simulink model "singlcontact_control_smc_lqr_mydimes_reaction"  (R2024a)
settings: Solver=VariableStepAuto  StartTime=0.0  StopTime=10  FixedStep=0.001  RelTol=1e-3
values from neighbouring files (symbols this model uses):
  ankle_servo_kd = 8    [robotParametersCtrl_mydiem_block_zmp.m]    (also in robotParametersCtrl_quad_modify_mydiem.m; robotParametersCtrl_quad_modify_mydiem_reaction.m)
  ankle_servo_ki = 4    [robotParametersCtrl_mydiem_block_zmp.m]    (also in robotParametersCtrl_quad_modify_mydiem.m; robotParametersCtrl_quad_modify_mydiem_reaction.m)
  ankle_servo_kp = 20    [robotParametersCtrl_mydiem_block_zmp.m]    (also in robotParametersCtrl_quad_modify_mydiem.m; robotParametersCtrl_quad_modify_mydiem_reaction.m)
  deriv_filter_coeff = 100    [robotParametersCtrl_mydiem_block_zmp.m]    (also in robotParametersCtrl_quad_modify_mydiem.m; robotParametersCtrl_quad_modify_mydiem_reaction.m)
  filter_coefficent_pid = 100    [robotParametersCtrl_mydiem_block_zmp.m]    (also in robotParametersCtrl_quad_modify_mydiem.m; robotParametersCtrl_quad_modify_mydiem_reaction.m)
  filter_coefficent_pids = 100    [robotParametersCtrl_quad_modify_mydiem_reaction.m]
  foot_z = 1.5    [robotParametersCtrl_mydiem_block_zmp.m]    (also in robotParametersCtrl_quad_modify_mydiem.m; robotParametersCtrl_quad_modify_mydiem_reaction.m)
  g = 9.81    [ABCDvalues_lqr_quad_mydime_reaction.m]    (also in robotParametersCtrl_mydiem_block_zmp.m = 9.80665; robotParametersCtrl_quad_modify_mydiem.m = 9.80665; robotParametersCtrl_quad_modify_mydiem_reaction.m = 9.80665)
  h = 32    [robotParametersCtrl_mydiem_block_zmp.m]    (also in robotParametersCtrl_quad_modify_mydiem.m; robotParametersCtrl_quad_modify_mydiem_reaction.m)
  height_plane = 0.025    [robotParametersCtrl_mydiem_block_zmp.m]    (also in robotParametersCtrl_quad_modify_mydiem.m; robotParametersCtrl_quad_modify_mydiem_reaction.m)
  hip_pitch_deriv = 20    [robotParametersCtrl_mydiem_block_zmp.m]    (also in robotParametersCtrl_quad_modify_mydiem.m = 200; robotParametersCtrl_quad_modify_mydiem_reaction.m = 200)
  hip_pitch_derivs = 200    [robotParametersCtrl_quad_modify_mydiem_reaction.m]
  hip_pitch_int = 0    [robotParametersCtrl_mydiem_block_zmp.m]    (also in robotParametersCtrl_quad_modify_mydiem.m = 150; robotParametersCtrl_quad_modify_mydiem_reaction.m = 150)
  hip_pitch_ints = 1500    [robotParametersCtrl_quad_modify_mydiem_reaction.m]
  hip_pitch_prop = 10    [robotParametersCtrl_mydiem_block_zmp.m]    (also in robotParametersCtrl_quad_modify_mydiem.m = 500; robotParametersCtrl_quad_modify_mydiem_reaction.m = 500)
  hip_pitch_props = 500    [robotParametersCtrl_quad_modify_mydiem_reaction.m]
  hip_roll_deriv = 28    [robotParametersCtrl_mydiem_block_zmp.m]    (also in robotParametersCtrl_quad_modify_mydiem.m = 280; robotParametersCtrl_quad_modify_mydiem_reaction.m = 280)
  hip_roll_derivs = 280    [robotParametersCtrl_quad_modify_mydiem_reaction.m]
  hip_roll_int = 0    [robotParametersCtrl_mydiem_block_zmp.m]    (also in robotParametersCtrl_quad_modify_mydiem.m = 180; robotParametersCtrl_quad_modify_mydiem_reaction.m = 180)
  hip_roll_ints = 180    [robotParametersCtrl_quad_modify_mydiem_reaction.m]
  hip_roll_prop = 10    [robotParametersCtrl_mydiem_block_zmp.m]    (also in robotParametersCtrl_quad_modify_mydiem.m = 300; robotParametersCtrl_quad_modify_mydiem_reaction.m = 300)
  hip_roll_props = 300    [robotParametersCtrl_quad_modify_mydiem_reaction.m]
  hip_servo_kd = 20    [robotParametersCtrl_mydiem_block_zmp.m]    (also in robotParametersCtrl_quad_modify_mydiem.m; robotParametersCtrl_quad_modify_mydiem_reaction.m)
  hip_servo_ki = 10    [robotParametersCtrl_mydiem_block_zmp.m]    (also in robotParametersCtrl_quad_modify_mydiem.m; robotParametersCtrl_quad_modify_mydiem_reaction.m)
  hip_servo_kp = 60    [robotParametersCtrl_mydiem_block_zmp.m]    (also in robotParametersCtrl_quad_modify_mydiem.m; robotParametersCtrl_quad_modify_mydiem_reaction.m)
  hip_smc_lamda = 85    [robotParametersCtrl_mydiem_block_zmp.m]    (also in robotParametersCtrl_quad_modify_mydiem.m; robotParametersCtrl_quad_modify_mydiem_reaction.m = 95)
  hip_smc_lamdas = 85    [robotParametersCtrl_quad_modify_mydiem_reaction.m]
  hip_smc_new = 25    [robotParametersCtrl_mydiem_block_zmp.m]    (also in robotParametersCtrl_quad_modify_mydiem.m; robotParametersCtrl_quad_modify_mydiem_reaction.m = 45)
  hip_smc_news = 25    [robotParametersCtrl_quad_modify_mydiem_reaction.m]
  init_angs_L = init_angs_R    [robotParametersCtrl_mydiem_block_zmp.m]    (also in robotParametersCtrl_quad_modify_mydiem.m; robotParametersCtrl_quad_modify_mydiem_reaction.m)
  init_angs_R = [0 -sum(init_angs) init_angs(2) 0 init_angs(1)]    [robotParametersCtrl_mydiem_block_zmp.m]    (also in robotParametersCtrl_quad_modify_mydiem.m; robotParametersCtrl_quad_modify_mydiem_reaction.m)
  init_height = h +                torso_z/2 + torso_offset_z + height_plane/2    (= 39.5125)    [robotParametersCtrl_mydiem_block_zmp.m]    (also in robotParametersCtrl_quad_modify_mydiem.m; robotParametersCtrl_quad_modify_mydiem_reaction.m)
  K = lqr(A, B, Q, R)    [ABCDvalues_lqr_quad_mydime_reaction.m]
  knee_pitch_deriv = 10    [robotParametersCtrl_mydiem_block_zmp.m]    (also in robotParametersCtrl_quad_modify_mydiem.m = 100; robotParametersCtrl_quad_modify_mydiem_reaction.m = 100)
  knee_pitch_derivs = 180    [robotParametersCtrl_quad_modify_mydiem_reaction.m]
  knee_pitch_int = 0    [robotParametersCtrl_mydiem_block_zmp.m]    (also in robotParametersCtrl_quad_modify_mydiem.m = 300; robotParametersCtrl_quad_modify_mydiem_reaction.m = 300)
  knee_pitch_ints = 7500    [robotParametersCtrl_quad_modify_mydiem_reaction.m]
  knee_pitch_prop = 10    [robotParametersCtrl_mydiem_block_zmp.m]    (also in robotParametersCtrl_quad_modify_mydiem.m = 400; robotParametersCtrl_quad_modify_mydiem_reaction.m = 400)
  knee_pitch_props = 1200    [robotParametersCtrl_quad_modify_mydiem_reaction.m]
  knee_servo_kd = 10    [robotParametersCtrl_mydiem_block_zmp.m]    (also in robotParametersCtrl_quad_modify_mydiem.m; robotParametersCtrl_quad_modify_mydiem_reaction.m)
  knee_servo_ki = 5    [robotParametersCtrl_mydiem_block_zmp.m]    (also in robotParametersCtrl_quad_modify_mydiem.m; robotParametersCtrl_quad_modify_mydiem_reaction.m)
  knee_servo_kp = 60    [robotParametersCtrl_mydiem_block_zmp.m]    (also in robotParametersCtrl_quad_modify_mydiem.m; robotParametersCtrl_quad_modify_mydiem_reaction.m)
  knee_smc_lamda = 140    [robotParametersCtrl_mydiem_block_zmp.m]    (also in robotParametersCtrl_quad_modify_mydiem.m; robotParametersCtrl_quad_modify_mydiem_reaction.m = 150)
  knee_smc_lamdas = 100    [robotParametersCtrl_quad_modify_mydiem_reaction.m]
  knee_smc_new = 80    [robotParametersCtrl_mydiem_block_zmp.m]    (also in robotParametersCtrl_quad_modify_mydiem.m; robotParametersCtrl_quad_modify_mydiem_reaction.m)
  knee_smc_news = 60    [robotParametersCtrl_quad_modify_mydiem_reaction.m]
  Kwalk = 0.6    [robotParametersCtrl_mydiem_block_zmp.m]    (also in robotParametersCtrl_quad_modify_mydiem.m; robotParametersCtrl_quad_modify_mydiem_reaction.m)
  l1 = 0.20    (= 0.2)    [ABCDvalues_lqr_quad_mydime_reaction.m]
  l2 = 0.20    (= 0.2)    [ABCDvalues_lqr_quad_mydime_reaction.m]
  lower_leg_length = 20    [robotParametersCtrl_mydiem_block_zmp.m]    (also in robotParametersCtrl_quad_modify_mydiem.m; robotParametersCtrl_quad_modify_mydiem_reaction.m)
  m1 = 0.45    [ABCDvalues_lqr_quad_mydime_reaction.m]
  m2 = 0.065    [ABCDvalues_lqr_quad_mydime_reaction.m]
  max_torque = 20    [robotParametersCtrl_mydiem_block_zmp.m]    (also in robotParametersCtrl_quad_modify_mydiem.m; robotParametersCtrl_quad_modify_mydiem_reaction.m)
  motion_time_constant = 0.01    [robotParametersCtrl_mydiem_block_zmp.m]    (also in robotParametersCtrl_quad_modify_mydiem.m; robotParametersCtrl_quad_modify_mydiem_reaction.m)
  plane_x = 25    [robotParametersCtrl_mydiem_block_zmp.m]    (also in robotParametersCtrl_quad_modify_mydiem.m; robotParametersCtrl_quad_modify_mydiem_reaction.m)
  plane_y = 3    [robotParametersCtrl_mydiem_block_zmp.m]    (also in robotParametersCtrl_quad_modify_mydiem.m; robotParametersCtrl_quad_modify_mydiem_reaction.m)
  stepHeight = 0.4    [ABCDvalues_lqr_quad_mydime_reaction.m]
  torso_offset_x = 17    [robotParametersCtrl_mydiem_block_zmp.m]    (also in robotParametersCtrl_quad_modify_mydiem.m; robotParametersCtrl_quad_modify_mydiem_reaction.m)
  torso_offset_x1 = -17    [robotParametersCtrl_mydiem_block_zmp.m]    (also in robotParametersCtrl_quad_modify_mydiem.m; robotParametersCtrl_quad_modify_mydiem_reaction.m)
  torso_offset_z = 0    [robotParametersCtrl_mydiem_block_zmp.m]    (also in robotParametersCtrl_quad_modify_mydiem.m; robotParametersCtrl_quad_modify_mydiem_reaction.m)
  torso_x = 40    [robotParametersCtrl_mydiem_block_zmp.m]    (also in robotParametersCtrl_quad_modify_mydiem.m; robotParametersCtrl_quad_modify_mydiem_reaction.m)
  torso_y = 20    [robotParametersCtrl_mydiem_block_zmp.m]    (also in robotParametersCtrl_quad_modify_mydiem.m; robotParametersCtrl_quad_modify_mydiem_reaction.m)
  torso_z = 15    [robotParametersCtrl_mydiem_block_zmp.m]    (also in robotParametersCtrl_quad_modify_mydiem.m; robotParametersCtrl_quad_modify_mydiem_reaction.m)
  Ts = 0.05    [ABCDvalues_lqr_quad_mydime_reaction.m]
  TsCtrl = 0.05    [robotParametersCtrl_mydiem_block_zmp.m]    (also in robotParametersCtrl_quad_modify_mydiem.m; robotParametersCtrl_quad_modify_mydiem_reaction.m)
  tWalk = 0.3    [robotParametersCtrl_mydiem_block_zmp.m]    (also in robotParametersCtrl_quad_modify_mydiem.m; robotParametersCtrl_quad_modify_mydiem_reaction.m)
  upper_leg_length = 20    [robotParametersCtrl_mydiem_block_zmp.m]    (also in robotParametersCtrl_quad_modify_mydiem.m; robotParametersCtrl_quad_modify_mydiem_reaction.m)
undefined symbols (not defined in the file or in its folder): X, Y, Z
libraries: simulink_extras x256, slpidlib x128, sm_lib x71, simulink x43, nesl_utility x35, walkingRobotUtils x21, dspsrcs4 x18, dspobslib x8
(part 1 of 33)
settings Model: Creator=sunil kumar  LastModifiedBy=USER
settings OptimizationCC: BlockReduction=off  DefaultParameterBehavior=Inlined  BufferReuse=off
settings RTWCC: GPUComputeCapability=3.5

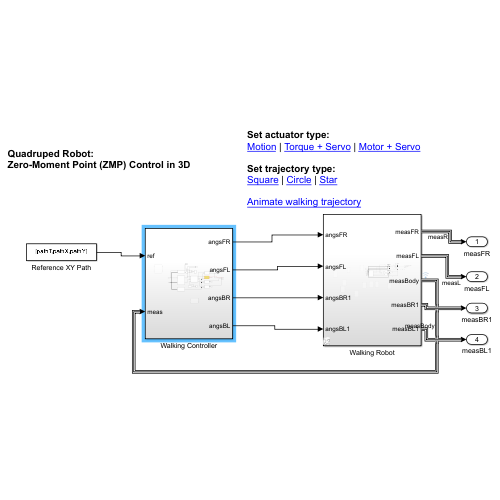
[thumbnail: Simulink's stored preview of the top-level diagram]
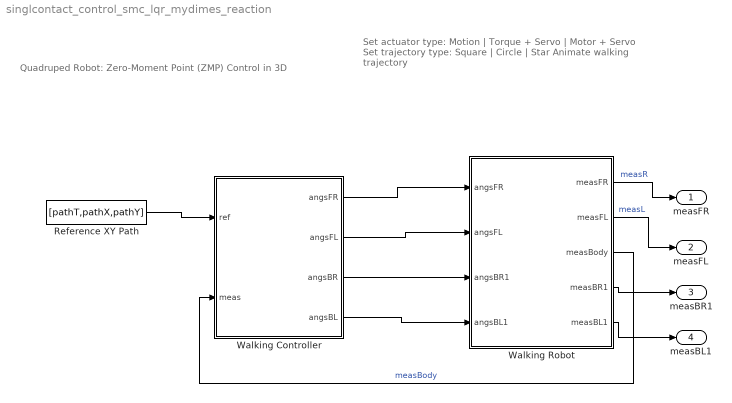
== system singlcontact_control_smc_lqr_mydimes_reaction ==
  note: Set actuator type:
      | Motion | Torque + Servo | Motor + Servo
      |
      | Set trajectory type:
      | Square | Circle | Star
      |
      | Animate walking trajectory
  note: Quadruped Robot:
      | Zero-Moment Point (ZMP) Control in 3D
  Reference XY Path : FromWorkspace  VariableName=[pathT,pathX,pathY]  SampleTime=TsCtrl  OutputAfterFinalValue=Holding final value
  Walking Controller : Subsystem
  Walking Robot : Subsystem  AncestorBlock=|
      | walkingRobotUtils/Walking Robot
      | (Control Design)
  measFR : Outport  VectorParamsAs1DForOutWhenUnconnected=off
  measFL : Outport  Port=2  VectorParamsAs1DForOutWhenUnconnected=off
  measBR1 : Outport  Port=3  VectorParamsAs1DForOutWhenUnconnected=off
  measBL1 : Outport  Port=4  VectorParamsAs1DForOutWhenUnconnected=off
  wires:
  Reference XY Path/1 -> Walking Controller/1(ref)
  Walking Robot/2(measFL) -> measFL/1  "measL"
  Walking Robot/1(measFR) -> measFR/1  "measR"
  Walking Controller/1(angsFR) -> Walking Robot/1(angsFR)
  Walking Controller/2(angsFL) -> Walking Robot/2(angsFL)
  Walking Robot/3(measBody) -> Walking Controller/2(meas)  "measBody"
  Walking Controller/3(angsBR) -> Walking Robot/3(angsBR1)
  Walking Controller/4(angsBL) -> Walking Robot/4(angsBL1)
  Walking Robot/4(measBR1) -> measBR1/1
  Walking Robot/5(measBL1) -> measBL1/1

== system singlcontact_control_smc_lqr_mydimes_reaction/Walking Controller ==
  ref : Inport
  meas : Inport  Port=2
  Calculate Attitude : Subsystem
  Digital Clock : DigitalClock  SampleTime=0.05
  Left Leg Inverse Kinematics : walkingRobotUtils/Inverse Kinematics (Control Design)  SystemSampleTime=-1  VariantActivationTime=update diagram  AllowFlexibleInterface=on  Latency=0  AutoFrameSizeCalculation=off
  Left Leg Inverse Kinematics1 : walkingRobotUtils/Inverse Kinematics (Control Design)  SystemSampleTime=-1  VariantActivationTime=update diagram  AllowFlexibleInterface=on  Latency=0  AutoFrameSizeCalculation=off
  Mux : Mux  Inputs=2
  Package Signals : Subsystem
  Position1 : Scope
  Right Leg Inverse Kinematics : walkingRobotUtils/Inverse Kinematics (Control Design)  SystemSampleTime=-1  VariantActivationTime=update diagram  AllowFlexibleInterface=on  Latency=0  AutoFrameSizeCalculation=off
  Right Leg Inverse Kinematics1 : walkingRobotUtils/Inverse Kinematics (Control Design)  SystemSampleTime=-1  VariantActivationTime=update diagram  AllowFlexibleInterface=on  Latency=0  AutoFrameSizeCalculation=off
  Scope : Scope  NumInputPorts=2
  Scope1 : Scope  NumInputPorts=4
  Scope2 : Scope
  Scope3 : Scope  NumInputPorts=2
  Step Planning Logic : Stateflow chart  Commented=on  TreatAsAtomicUnit=on
  ZMP Controller : Subsystem
  Zero-Order Hold : ZeroOrderHold  SampleTime=0.005
  final logic working quad_trot : MATLAB Function  TreatAsAtomicUnit=on
  final logic working quad_walk1 : MATLAB Function  Commented=on  TreatAsAtomicUnit=on
  angsFR : Outport  VectorParamsAs1DForOutWhenUnconnected=off
  angsFL : Outport  Port=2  VectorParamsAs1DForOutWhenUnconnected=off
  angsBR : Outport  Port=3  VectorParamsAs1DForOutWhenUnconnected=off
  angsBL : Outport  Port=4  VectorParamsAs1DForOutWhenUnconnected=off
  wires:
  ref/1 -> ZMP Controller/1(ref), Package Signals/1(ref)
  Right Leg Inverse Kinematics/1 -> Scope1/1, angsFR/1
  Left Leg Inverse Kinematics/1 -> Scope1/3, angsFL/1
  meas/1 -> Calculate Attitude/1(meas), Package Signals/2(meas), ZMP Controller/2("meas ")
  Package Signals/2(y) -> Zero-Order Hold/1  "Y"
  Package Signals/1(x) -> Scope3/1, Mux/1  "X"
  Calculate Attitude/1(att) -> Left Leg Inverse Kinematics/2, Right Leg Inverse Kinematics1/2, Right Leg Inverse Kinematics/2, Left Leg Inverse Kinematics1/2
  Digital Clock/1 -> final logic working quad_trot/3(timeElapsed), Scope2/1
  final logic working quad_trot/1(footFR) -> Right Leg Inverse Kinematics/1
  ZMP Controller/1(stepFwd) -> final logic working quad_trot/1(stepFwd), Scope/1
  ZMP Controller/2(stepLat) -> final logic working quad_trot/2(stepLat), Scope/2
  final logic working quad_trot/2(footFL) -> Left Leg Inverse Kinematics/1  "L"
  final logic working quad_trot/4(footBL) -> Left Leg Inverse Kinematics1/1
  final logic working quad_trot/3(footBR) -> Right Leg Inverse Kinematics1/1
  Right Leg Inverse Kinematics1/1 -> Scope1/2, angsBR/1
  Left Leg Inverse Kinematics1/1 -> Scope1/4, angsBL/1
  Zero-Order Hold/1 -> Scope3/2, Mux/2
  Mux/1 -> Position1/1

== system singlcontact_control_smc_lqr_mydimes_reaction/Walking Robot ==
  angsFR : Inport
  angsFL : Inport  Port=2
  angsBR1 : Inport  Port=3
  angsBL1 : Inport  Port=4
  6-DOF Joint : sm_lib/Joints/6-DOF Joint  JointMode=Normal  CompositeWrenchDir=FollowerOnBase  CompositeWrenchFrame=BaseFrame  SenseConstraintForce=off  SenseConstraintTorque=off  SenseTotalForce=off  SenseTotalTorque=off  PxPositionTargetSpecify=on  PxPositionTargetPriority=High  PxPositionTargetValue=0  PxPositionTargetValueUnits=m  PxVelocityTargetSpecify=off  PxVelocityTargetPriority=High  PxVelocityTargetValue=0  PxVelocityTargetValueUnits=m/s  PxEquilibriumPosition=0  PxEquilibriumPositionUnits=m  PxSpringStiffness=0  PxSpringStiffnessUnits=N/m  PxDampingCoefficient=world_damping  PxDampingCoefficientUnits=N/(m/s)  PxLowerLimitSpecify=off  PxLowerLimitBound=-1  PxLowerLimitBoundUnits=m  PxLowerLimitStiffness=1e6  PxLowerLimitStiffnessUnits=N/m  PxLowerLimitDamping=1e3  PxLowerLimitDampingUnits=N/(m/s)  PxLowerLimitTransitionRegionWidth=1e-4  PxLowerLimitTransitionRegionWidthUnits=m  PxUpperLimitSpecify=off  PxUpperLimitBound=1  PxUpperLimitBoundUnits=m  PxUpperLimitStiffness=1e6  PxUpperLimitStiffnessUnits=N/m  PxUpperLimitDamping=1e3  PxUpperLimitDampingUnits=N/(m/s)  PxUpperLimitTransitionRegionWidth=1e-4  PxUpperLimitTransitionRegionWidthUnits=m  PxTorqueActuationMode=NoTorque  PxMotionActuationMode=ComputedMotion  PxSensePosition=off  PxSenseVelocity=off  PxSenseAcceleration=off  PxSenseTorqueForce=off  PxSenseLowerLimitTorqueForce=off  PxSenseUpperLimitTorqueForce=off  PyPositionTargetSpecify=on  PyPositionTargetPriority=High  PyPositionTargetValue=0  PyPositionTargetValueUnits=m  PyVelocityTargetSpecify=off  PyVelocityTargetPriority=High  PyVelocityTargetValue=0  PyVelocityTargetValueUnits=m/s  PyEquilibriumPosition=0  PyEquilibriumPositionUnits=m  PySpringStiffness=0  PySpringStiffnessUnits=N/m  PyDampingCoefficient=world_damping  PyDampingCoefficientUnits=N/(m/s)  PyLowerLimitSpecify=off  PyLowerLimitBound=-1  PyLowerLimitBoundUnits=m  PyLowerLimitStiffness=1e6  PyLowerLimitStiffnessUnits=N/m  PyLowerLimitDamping=1e3  PyLowerLimitDampingUnits=N/(m/s)  PyLowerLimitTransitionRegionWidth=1e-4  PyLowerLimitTransitionRegionWidthUnits=m  PyUpperLimitSpecify=off  PyUpperLimitBound=1  PyUpperLimitBoundUnits=m  PyUpperLimitStiffness=1e6  PyUpperLimitStiffnessUnits=N/m  PyUpperLimitDamping=1e3  PyUpperLimitDampingUnits=N/(m/s)  PyUpperLimitTransitionRegionWidth=1e-4  PyUpperLimitTransitionRegionWidthUnits=m  PyTorqueActuationMode=NoTorque  PyMotionActuationMode=ComputedMotion  PySensePosition=off  PySenseVelocity=off  PySenseAcceleration=off  PySenseTorqueForce=off  PySenseLowerLimitTorqueForce=off  PySenseUpperLimitTorqueForce=off  PzPositionTargetSpecify=on  PzPositionTargetPriority=High  PzPositionTargetValue=init_height  PzPositionTargetValueUnits=cm  PzVelocityTargetSpecify=off  PzVelocityTargetPriority=High  PzVelocityTargetValue=0  PzVelocityTargetValueUnits=m/s  PzEquilibriumPosition=0  PzEquilibriumPositionUnits=m  PzSpringStiffness=0  PzSpringStiffnessUnits=N/m  PzDampingCoefficient=world_damping  PzDampingCoefficientUnits=N/(m/s)  PzLowerLimitSpecify=off  PzLowerLimitBound=-1  PzLowerLimitBoundUnits=m  PzLowerLimitStiffness=1e6  PzLowerLimitStiffnessUnits=N/m  PzLowerLimitDamping=1e3  PzLowerLimitDampingUnits=N/(m/s)  PzLowerLimitTransitionRegionWidth=1e-4  PzLowerLimitTransitionRegionWidthUnits=m  PzUpperLimitSpecify=off  PzUpperLimitBound=1  PzUpperLimitBoundUnits=m  PzUpperLimitStiffness=1e6  PzUpperLimitStiffnessUnits=N/m  PzUpperLimitDamping=1e3  PzUpperLimitDampingUnits=N/(m/s)  PzUpperLimitTransitionRegionWidth=1e-4  PzUpperLimitTransitionRegionWidthUnits=m  PzTorqueActuationMode=NoTorque  PzMotionActuationMode=ComputedMotion  PzSensePosition=off  PzSenseVelocity=off  PzSenseAcceleration=off  PzSenseTorqueForce=off  PzSenseLowerLimitTorqueForce=off  PzSenseUpperLimitTorqueForce=off  SphPositionTargetSpecify=off  SphPositionTargetPriority=High  SphPositionTargetRotationMethod=None  SphPositionTargetFollAlignAxisA=+X  SphPositionTargetBaseAlignAxisA=+Y  SphPositionTargetFollAlignAxisB=+Y  SphPositionTargetBaseAlignAxisB=+Z  SphPositionTargetRotationStandardAxis=+Z  SphPositionTargetRotationAngle=0.0  SphPositionTargetRotationAngleUnits=deg  SphPositionTargetRotationArbitraryAxis=[0 0 1]  SphPositionTargetRotationSequenceAxes=FollowerAxes  SphPositionTargetRotationSequence=XYX  SphPositionTargetRotationSequenceAngles=[0 0 0]  SphPositionTargetRotationSequenceAnglesUnits=deg  SphPositionTargetRotationMatrix=eye(3)  SphPositionTargetQuaternion=[1 0 0 0]  SphVelocityTargetSpecify=off  SphVelocityTargetPriority=High  SphVelocityTargetValue=[0 0 0]  SphVelocityTargetValueUnits=deg/s  SphVelocityTargetInFollowerFrame=on  SphEqPosRotationMethod=None  SphEqPosFollAlignAxisA=+X  SphEqPosBaseAlignAxisA=+Y  SphEqPosFollAlignAxisB=+Y  SphEqPosBaseAlignAxisB=+Z  SphEqPosRotationStandardAxis=+Z  SphEqPosRotationAngle=0.0  SphEqPosRotationAngleUnits=deg  SphEqPosRotationArbitraryAxis=[0 0 1]  SphEqPosRotationSequenceAxes=FollowerAxes  SphEqPosRotationSequence=XYX  SphEqPosRotationSequenceAngles=[0 0 0]  SphEqPosRotationSequenceAnglesUnits=deg  SphEqPosRotationMatrix=[1 0 0; 0 1 0; 0 0 1]  SphEqPosQuaternion=[1 0 0 0]  SphSpringStiffness=0  SphSpringStiffnessUnits=N*m/deg  SphDampingCoefficient=world_rot_damping  SphDampingCoefficientUnits=N*m/(rad/s)  SphLowerLimitSpecify=off  SphLowerLimitBound=15  SphLowerLimitBoundUnits=deg  SphLowerLimitStiffness=1e4  SphLowerLimitStiffnessUnits=N*m/deg  SphLowerLimitDamping=10  SphLowerLimitDampingUnits=N*m/(deg/s)  SphLowerLimitTransitionRegionWidth=0.1  SphLowerLimitTransitionRegionWidthUnits=deg  SphUpperLimitSpecify=off  SphUpperLimitBound=45  SphUpperLimitBoundUnits=deg  SphUpperLimitStiffness=1e4  SphUpperLimitStiffnessUnits=N*m/deg  SphUpperLimitDamping=10  SphUpperLimitDampingUnits=N*m/(deg/s)  SphUpperLimitTransitionRegionWidth=0.1  SphUpperLimitTransitionRegionWidthUnits=deg  SphTorqueActuationMode=NoTorque  SphActuateTorqueX=off  SphActuateTorqueY=off  SphActuateTorqueZ=off  SphActuateTorque=off  SphActuationFrame=BaseFrame  SphSensePosition=off  SphSenseVelocityX=off  SphSenseVelocityY=off  SphSenseVelocityZ=off  SphSenseVelocity=off  SphSenseAccelerationX=off  SphSenseAccelerationY=off  SphSenseAccelerationZ=off  SphSenseAcceleration=off  SphSenseLowerLimitTorqueMag=off  SphSenseUpperLimitTorqueMag=off  SphSensingFrame=BaseFrame
  Left Hip to Torso : sm_lib/Frames and Transforms/Rigid Transform  RotationMethod=None  FollAlignAxisA=+X  BaseAlignAxisA=+Y  FollAlignAxisB=+Y  BaseAlignAxisB=+Z  RotationStandardAxis=+Z  RotationAngle=0.0  RotationAngleUnits=deg  RotationArbitraryAxis=[0 0 1]  RotationSequenceAxes=FollowerAxes  RotationSequence=XYX  RotationSequenceAngles=[0 0 0]  RotationSequenceAnglesUnits=deg  RotationMatrix=[1 0 0; 0 1 0; 0 0 1]  Quaternion=[1 0 0 0]  TranslationMethod=Cartesian  TranslationCartesianOffset=[torso_offset_x torso_y/2 torso_offset_z]  TranslationCartesianOffsetUnits=cm  TranslationStandardAxis=+Z  TranslationStandardOffset=0  TranslationStandardOffsetUnits=cm  TranslationROffset=0  TranslationROffsetUnits=m  TranslationThetaOffset=0  TranslationThetaOffsetUnits=deg  TranslationZOffset=0  TranslationZOffsetUnits=m
  Left Hip to Torso1 : sm_lib/Frames and Transforms/Rigid Transform  RotationMethod=None  FollAlignAxisA=+X  BaseAlignAxisA=+Y  FollAlignAxisB=+Y  BaseAlignAxisB=+Z  RotationStandardAxis=+Z  RotationAngle=0.0  RotationAngleUnits=deg  RotationArbitraryAxis=[0 0 1]  RotationSequenceAxes=FollowerAxes  RotationSequence=XYX  RotationSequenceAngles=[0 0 0]  RotationSequenceAnglesUnits=deg  RotationMatrix=[1 0 0; 0 1 0; 0 0 1]  Quaternion=[1 0 0 0]  TranslationMethod=Cartesian  TranslationCartesianOffset=[torso_offset_x1 torso_y/2 torso_offset_z]  TranslationCartesianOffsetUnits=cm  TranslationStandardAxis=+Z  TranslationStandardOffset=0  TranslationStandardOffsetUnits=cm  TranslationROffset=0  TranslationROffsetUnits=m  TranslationThetaOffset=0  TranslationThetaOffsetUnits=deg  TranslationZOffset=0  TranslationZOffsetUnits=m
  Lqr+Lqr+reaction : Subsystem  Commented=on  VariantControl=actuatorType == 1
  NO CONTROLLER : Subsystem  Commented=on  VariantControl=actuatorType == 1
  PS-Simulink Converter : nesl_utility/PS-Simulink Converter  PhysicalDomain=network_engine_domain  SubClassName=ps_output  LeftPortType=input  RightPortType=output  PseudoPeriodic=off  Frequencies=[]  VectorFormat=inherit  Unit=inherit  AffineConversion=off
  PS-Simulink Converter1 : nesl_utility/PS-Simulink Converter  PhysicalDomain=network_engine_domain  SubClassName=ps_output  LeftPortType=input  RightPortType=output  PseudoPeriodic=off  Frequencies=[]  VectorFormat=inherit  Unit=inherit  AffineConversion=off
  PS-Simulink Converter2 : nesl_utility/PS-Simulink Converter  PhysicalDomain=network_engine_domain  SubClassName=ps_output  LeftPortType=input  RightPortType=output  PseudoPeriodic=off  Frequencies=[]  VectorFormat=inherit  Unit=inherit  AffineConversion=off
  Pid+Pid+reaction1 : Subsystem  Commented=on  VariantControl=actuatorType == 1
  Right Hip to Torso : sm_lib/Frames and Transforms/Rigid Transform  RotationMethod=None  FollAlignAxisA=+X  BaseAlignAxisA=+Y  FollAlignAxisB=+Y  BaseAlignAxisB=+Z  RotationStandardAxis=+Z  RotationAngle=0.0  RotationAngleUnits=deg  RotationArbitraryAxis=[0 0 1]  RotationSequenceAxes=FollowerAxes  RotationSequence=XYX  RotationSequenceAngles=[0 0 0]  RotationSequenceAnglesUnits=deg  RotationMatrix=[1 0 0; 0 1 0; 0 0 1]  Quaternion=[1 0 0 0]  TranslationMethod=Cartesian  TranslationCartesianOffset=[torso_offset_x -torso_y/2 torso_offset_z]  TranslationCartesianOffsetUnits=cm  TranslationStandardAxis=+Z  TranslationStandardOffset=0  TranslationStandardOffsetUnits=cm  TranslationROffset=0  TranslationROffsetUnits=m  TranslationThetaOffset=0  TranslationThetaOffsetUnits=deg  TranslationZOffset=0  TranslationZOffsetUnits=m
  Right Hip to Torso1 : sm_lib/Frames and Transforms/Rigid Transform  RotationMethod=None  FollAlignAxisA=+X  BaseAlignAxisA=+Y  FollAlignAxisB=+Y  BaseAlignAxisB=+Z  RotationStandardAxis=+Z  RotationAngle=0.0  RotationAngleUnits=deg  RotationArbitraryAxis=[0 0 1]  RotationSequenceAxes=FollowerAxes  RotationSequence=XYX  RotationSequenceAngles=[0 0 0]  RotationSequenceAnglesUnits=deg  RotationMatrix=[1 0 0; 0 1 0; 0 0 1]  Quaternion=[1 0 0 0]  TranslationMethod=Cartesian  TranslationCartesianOffset=[torso_offset_x1 -torso_y/2 torso_offset_z]  TranslationCartesianOffsetUnits=cm  TranslationStandardAxis=+Z  TranslationStandardOffset=0  TranslationStandardOffsetUnits=cm  TranslationROffset=0  TranslationROffsetUnits=m  TranslationThetaOffset=0  TranslationThetaOffsetUnits=deg  TranslationZOffset=0  TranslationZOffsetUnits=m
  Robot Joint Controller : Subsystem  Commented=on  Variant=on
  Robot Leg BL3 : Subsystem
  Robot Leg BR2 : Subsystem
  Robot Leg FL1 : Subsystem
  Robot Leg FR : Subsystem
  Scope : Scope  NumInputPorts=2
  Sensors : Subsystem
  Torso : sm_lib/Body Elements/Brick Solid  BrickDimensions=[torso_x torso_y torso_z]  BrickDimensionsUnits=cm  ExportEntireGeometry=off  InertiaType=PointMass  BasedOnType=Mass  Density=density  DensityUnits=kg/m^3  Mass=6  MassUnits=kg  CenterOfMass=[0 0 0]  CenterOfMassUnits=m  MomentsOfInertia=[1 1 1]  MomentsOfInertiaUnits=kg*m^2  ProductsOfInertia=[1 1 1]  ProductsOfInertiaUnits=kg*m^2  GraphicType=FromGeometry  MarkerShape=Sphere  MarkerSize=10  GraphicVisPropType=SimpleVisualProperties  GraphicDiffuseColor=[0.5 0.1 0.5]  GraphicOpacity=1.0  GraphicSpecularColor=[0.5 0.5 0.5 1.0]  GraphicAmbientColor=[0.15 0.15 0.15 1.0]  GraphicEmissiveColor=[0.0 0.0 0.0 1.0]  GraphicShininess=75  DoExposeReferenceFrame=on  SerializedFrames=<Frames><Frame><Id>Frame1</Id><Value><Name>F1</Name><Origin><Source>CenterOfMassFrame</Source><FeatureName></FeatureName></Origin><PrimaryAxis><DefinedDirection>+Z</DefinedDirection><Source>ReferenceFrame</Source><SourceDirection>+Z</SourceDirection><FeatureName></FeatureName></PrimaryAxis><SecondaryAxis><DefinedDirection>+Y</DefinedDirection><Source>ReferenceFrame</Source><SourceDirection>+X</SourceDirection><FeatureName></FeatureName></SecondaryAxis></Value></Frame></Frames>
  Torso2torso : sm_lib/Frames and Transforms/Rigid Transform  Commented=on  RotationMethod=None  FollAlignAxisA=+X  BaseAlignAxisA=+Y  FollAlignAxisB=+Y  BaseAlignAxisB=+Z  RotationStandardAxis=+Z  RotationAngle=0.0  RotationAngleUnits=deg  RotationArbitraryAxis=[0 0 1]  RotationSequenceAxes=FollowerAxes  RotationSequence=XYX  RotationSequenceAngles=[0 0 0]  RotationSequenceAnglesUnits=deg  RotationMatrix=[1 0 0; 0 1 0; 0 0 1]  Quaternion=[1 0 0 0]  TranslationMethod=Cartesian  TranslationCartesianOffset=[0 0 -7.5]  TranslationCartesianOffsetUnits=cm  TranslationStandardAxis=+Z  TranslationStandardOffset=0  TranslationStandardOffsetUnits=cm  TranslationROffset=0  TranslationROffsetUnits=m  TranslationThetaOffset=0  TranslationThetaOffsetUnits=deg  TranslationZOffset=0  TranslationZOffsetUnits=m
  Trajectory Display : sm_lib/Curves and Surfaces/Spline  DataPoints=interPts  DataPointsUnits=m  EndConditionType=Natural  GraphicType=FromGeometry  MarkerShape=Sphere  MarkerSize=10  GraphicVisPropType=SimpleVisualProperties  GraphicDiffuseColor=[0 0 0]  GraphicOpacity=1.0  GraphicSpecularColor=[0.5 0.5 0.5 1.0]  GraphicAmbientColor=[0.15 0.15 0.15 1.0]  GraphicEmissiveColor=[0.0 0.0 0.0 1.0]  GraphicShininess=75
  Transform Sensor : sm_lib/Frames and Transforms/Transform Sensor  MeasurementFrame=Base  RotationSequence=XYZ  SenseAngle=off  SenseAxis=off  SenseQ=off  SenseR=off  SenseRotationSequence=off  SenseOmegaX=off  SenseOmegaY=off  SenseOmegaZ=off  SenseOmega=off  SenseQDot=off  SenseRDot=off  SenseRotationSequenceDot=off  SenseAlphaX=off  SenseAlphaY=off  SenseAlphaZ=off  SenseAlpha=off  SenseQDDot=off  SenseRDDot=off  SenseX=on  SenseY=on  SenseZ=on  SenseXYZ=off  SenseRad=off  SenseAzim=off  SenseDist=off  SenseInc=off  SenseXDot=on  SenseYDot=off  SenseZDot=off  SenseXYZDot=off  SenseRadDot=off  SenseAzimDot=off  SenseDistDot=off  SenseIncDot=off  SenseXDDot=off  SenseYDDot=off  SenseZDDot=off  SenseXYZDDot=off  SenseRadDDot=off  SenseAzimDDot=off  SenseDistDDot=off  SenseIncDDot=off
  World and Ground : Subsystem
  XY Graph : Record  FileSettingsInternal="{\"entries\":[{\"content\":{\"excelSettings\":{\"content\":{},\"type\":\"Streamout.ExcelSettings\"}},\"type\":\"Streamout.FileSettingStorage\",\"uuid\":\"\"}],\"packageUris\":[\"http:\\/\\/schema.mathworks.com\\/mf0\\/streamout_blocks\\/R2020a\"],\"version\":\"1.0\"}"  Layout=[1 1]  SignalsInternal="{\"entries\":[{\"content\":{\"signals\":[{\"content\":{\"blockPath\":[],\"dimensions\":[1],\"domain\":\"\",\"lineColor\":\"#139fff\",\"lineWidth\":2,\"port\":1,\"sid\":[\"\"],\"signalID\":1,\"signalName\":\"PS-Simulink\\nConverter\"},\"type\":\"RecordBlkView.Signal\",\"uuid\":\"\"},{\"content\":{\"blockPath\":[],\"dimensions\":[1],\"domain\":\"\",\"lineColor\":\"#ff6929\",\"lineWidth\":2,\"port\":2,\"sid\":[\"\"],\"signalID\":2,\"signalName\":\"PS-Simulink\\nConverter1\"},\"type\":\"RecordBlkView.Signal\",\"uuid\":\"\"}]},\"type\":\"RecordBlkView.InputSignals\",\"uuid\":\"\"}],\"packageUris\":[\"http:\\/\\/schema.mathworks.com\\/mf0\\/streamout_blocks\\/R2020a\"],\"version\":\"1.0\"}"  CompatibilityTag=XY
  lqr + reaction+ CONTROL1 : Subsystem  Commented=on  VariantControl=actuatorType == 2
  lqr CONTROL : Subsystem  Commented=on  VariantControl=actuatorType == 2
  payload : sm_lib/Body Elements/Brick Solid  Commented=on  BrickDimensions=[10 15 10]  BrickDimensionsUnits=cm  ExportEntireGeometry=off  InertiaType=PointMass  BasedOnType=Mass  Density=density  DensityUnits=kg/m^3  Mass=1.2  MassUnits=kg  CenterOfMass=[0 0 0]  CenterOfMassUnits=m  MomentsOfInertia=[1 1 1]  MomentsOfInertiaUnits=kg*m^2  ProductsOfInertia=[1 1 1]  ProductsOfInertiaUnits=kg*m^2  GraphicType=FromGeometry  MarkerShape=Sphere  MarkerSize=10  GraphicVisPropType=SimpleVisualProperties  GraphicDiffuseColor=[0.5 0.5 0.5]  GraphicOpacity=1.0  GraphicSpecularColor=[0.5 0.5 0.5 1.0]  GraphicAmbientColor=[0.15 0.15 0.15 1.0]  GraphicEmissiveColor=[0.0 0.0 0.0 1.0]  GraphicShininess=75  DoExposeReferenceFrame=on  SerializedFrames=<Frames><Frame><Id>Frame1</Id><Value><Name>F1</Name><Origin><Source>CenterOfMassFrame</Source><FeatureName></FeatureName></Origin><PrimaryAxis><DefinedDirection>+Z</DefinedDirection><Source>ReferenceFrame</Source><SourceDirection>+Z</SourceDirection><FeatureName></FeatureName></PrimaryAxis><SecondaryAxis><DefinedDirection>+Y</DefinedDirection><Source>ReferenceFrame</Source><SourceDirection>+X</SourceDirection><FeatureName></FeatureName></SecondaryAxis></Value></Frame></Frames>
  pid : Subsystem  Commented=on  VariantControl=actuatorType == 2
  smc+lqr : Subsystem  Commented=on  VariantControl=actuatorType == 1
  smc+lqr+neuro1+reaction1 : Subsystem  VariantControl=actuatorType == 1
  smc+neuro+distur1 : Subsystem  Commented=on  VariantControl=actuatorType == 1
  smc+neuro1+reaction : Subsystem  Commented=on  VariantControl=actuatorType == 1
  smc+smcr+neuro1+reaction2 : Subsystem  Commented=on  VariantControl=actuatorType == 1
  measFR : Outport  VectorParamsAs1DForOutWhenUnconnected=off
  measFL : Outport  Port=2  VectorParamsAs1DForOutWhenUnconnected=off
  measBody : Outport  Port=3  VectorParamsAs1DForOutWhenUnconnected=off
  measBR1 : Outport  Port=4  VectorParamsAs1DForOutWhenUnconnected=off
  measBL1 : Outport  Port=5  VectorParamsAs1DForOutWhenUnconnected=off
  wires:
  Sensors/1(meas) -> measBody/1
  Robot Leg FR/1(meas) -> smc+lqr+neuro1+reaction1/3(measFR), measFR/1
  Robot Leg FL1/1(meas) -> smc+lqr+neuro1+reaction1/4(measFL), measFL/1
  smc+lqr+neuro1+reaction1/1(InputFR) -> Scope/2, Robot Leg FR/1(angs)
  smc+lqr+neuro1+reaction1/2(InputFL) -> Robot Leg FL1/1(angs)
  smc+lqr+neuro1+reaction1/3(InputBR) -> Robot Leg BR2/1(angs)
  smc+lqr+neuro1+reaction1/4(InputBL) -> Robot Leg BL3/1(angs)
  angsFR/1 -> Scope/1, smc+lqr+neuro1+reaction1/1(refFR)
  angsFL/1 -> smc+lqr+neuro1+reaction1/2(refFL)
  angsBR1/1 -> smc+lqr+neuro1+reaction1/7(refBR)
  angsBL1/1 -> smc+lqr+neuro1+reaction1/8(refBL)
  Robot Leg BR2/1(meas) -> smc+lqr+neuro1+reaction1/6(measBR), measBR1/1
  Robot Leg BL3/1(meas) -> smc+lqr+neuro1+reaction1/5(measBL), measBL1/1
  PS-Simulink Converter/1 -> XY Graph/1
  PS-Simulink Converter1/1 -> XY Graph/2
  PS-Simulink Converter2/1 -> ?
  connections:
  Robot Leg FL1/RConn2 -- World and Ground/RConn1 -- Robot Leg FR/RConn2 -- Robot Leg BL3/RConn2 -- Robot Leg BR2/RConn2
  6-DOF Joint/LConn1 -- Sensors/LConn1 -- Trajectory Display/LConn1 -- World and Ground/LConn1
  6-DOF Joint/RConn1 -- Left Hip to Torso1/LConn1 -- Right Hip to Torso1/LConn1 -- Left Hip to Torso/LConn1 -- Torso/RConn1 -- Sensors/RConn1 -- Right Hip to Torso/LConn1
  Robot Leg FL1/RConn1 -- Left Hip to Torso/RConn1
  Robot Leg FR/RConn1 -- Right Hip to Torso/RConn1
  Robot Leg BR2/RConn1 -- Right Hip to Torso1/RConn1
  Robot Leg BL3/RConn1 -- Left Hip to Torso1/RConn1
  Torso/LConn1 -- Transform Sensor/RConn1
  PS-Simulink Converter/LConn1 -- Transform Sensor/RConn2
  Transform Sensor/RConn3 -- PS-Simulink Converter1/LConn1
  PS-Simulink Converter2/LConn1 -- Transform Sensor/RConn4

== system singlcontact_control_smc_lqr_mydimes_reaction/Walking Controller/Calculate Attitude ==
  meas : Inport
  Bus Selector : BusSelector  OutputSignals=R
  Rotation Matrix to Roll Pitch Yaw : walkingRobotUtils/Rotation Matrix to  Roll Pitch Yaw  SystemSampleTime=-1  VariantActivationTime=update diagram  AllowFlexibleInterface=on  Latency=0  AutoFrameSizeCalculation=off
  att : Outport  VectorParamsAs1DForOutWhenUnconnected=off
  wires:
  Bus Selector/1 -> Rotation Matrix to Roll Pitch Yaw/1  "<R>"
  meas/1 -> Bus Selector/1
  Rotation Matrix to Roll Pitch Yaw/1 -> att/1

== system singlcontact_control_smc_lqr_mydimes_reaction/Walking Controller/Package Signals ==
  ref : Inport
  meas : Inport  Port=2
  Bus Selector : BusSelector  OutputSignals=X,Y
  Demux1 : Demux  Outputs=2
  Mux : Mux  Inputs=2
  Mux1 : Mux  Inputs=2
  x : Outport  VectorParamsAs1DForOutWhenUnconnected=off
  y : Outport  Port=2  VectorParamsAs1DForOutWhenUnconnected=off
  wires:
  ref/1 -> Demux1/1
  Demux1/1 -> Mux/1  "xref"
  Bus Selector/2 -> Mux1/2  "<Y>"
  Mux/1 -> x/1
  meas/1 -> Bus Selector/1
  Bus Selector/1 -> Mux/2  "<X>"
  Mux1/1 -> y/1
  Demux1/2 -> Mux1/1  "yref"

== system singlcontact_control_smc_lqr_mydimes_reaction/Walking Controller/ZMP Controller ==
  ref : Inport
  "meas " : Inport  Port=2
  Bus Selector : BusSelector  OutputSignals=X,Y,R
  Bus Selector1 : BusSelector  OutputSignals=AX,AY
  Demux : Demux  Outputs=2
  Log Step Lengths : Subsystem
  MATLAB Function1 : MATLAB Function  Commented=on  TreatAsAtomicUnit=on
  MATLAB Function3 : MATLAB Function  TreatAsAtomicUnit=on
  Mux1 : Mux  Inputs=2
  R : Scope
  Scope1 : Scope
  X Acceleration Filter : DiscreteTransferFcn  Numerator=[-1*0.02469]  Denominator=[1 -0.9753]
  Xmes : Scope
  Xref : Scope
  Y Acceleration Filter : DiscreteTransferFcn  Numerator=[-1*0.02469]  Denominator=[1 -0.9753]
  Ymes : Scope
  Yref : Scope
  accel_x : Scope
  accel_y : Scope
  original : MATLAB Function  Commented=on  TreatAsAtomicUnit=on
  stepFwd : Outport  VectorParamsAs1DForOutWhenUnconnected=off
  stepLat : Outport  Port=2  VectorParamsAs1DForOutWhenUnconnected=off
  wires:
  ref/1 -> Demux/1
  Demux/1 -> Mux1/1, MATLAB Function3/1(Xref), Xref/1  "Xref"
  Bus Selector/1 -> MATLAB Function3/3(Xmes), Xmes/1  "<X>"
  Bus Selector/2 -> MATLAB Function3/4(Ymes), Ymes/1  "<Y>"
  Demux/2 -> Mux1/2, MATLAB Function3/2(Yref), Yref/1  "Yref"
  Bus Selector/3 -> MATLAB Function3/7(R), R/1  "<R>"
  "meas "/1 -> Bus Selector1/1, Bus Selector/1
  Bus Selector1/1 -> X Acceleration Filter/1  "<AX>"
  Bus Selector1/2 -> Y Acceleration Filter/1  "<AY>"
  X Acceleration Filter/1 -> MATLAB Function3/5(accel_x), accel_x/1  "accel_x"
  Y Acceleration Filter/1 -> MATLAB Function3/6(accel_y), accel_y/1  "accel_y"
  MATLAB Function3/1(posoutx) -> stepFwd/1, Log Step Lengths/1(stepFwd)
  MATLAB Function3/2(posouty) -> Log Step Lengths/4(stepLat), stepLat/1
  Mux1/1 -> Scope1/1

== system singlcontact_control_smc_lqr_mydimes_reaction/Walking Robot/Lqr+Lqr+reaction ==
  refFR : Inport
  refFL : Inport  Port=2
  measFR : Inport  Port=3
  measFL : Inport  Port=4
  measBL : Inport  Port=5
  measBR : Inport  Port=6
  refBR : Inport  Port=7
  refBL : Inport  Port=8
  Demux{,1..6} (7 alike) : Demux  Outputs=3
  LQR Controllers FR : Subsystem
  LQR Controllers FR1 : Subsystem
  LQR Controllers FR2 : Subsystem
  LQR Controllers FR3 : Subsystem
  LQR2 Controllers BL : Subsystem
  LQR2 Controllers BR : Subsystem
  LQR2 Controllers FL : Subsystem
  LQR2 Controllers FR : Subsystem
  Lqr : Subsystem
  Mux : Mux  Inputs=2
  NOT : Logic  Operator=NOT  IconShape=distinctive  AllPortsSameDT=off  OutDataTypeStr=boolean
  SMC Controllers FR1 : Subsystem  Commented=on
  SMC Controllers FR2 : Subsystem  Commented=on
  SMC Controllers FR3 : Subsystem  Commented=on
  Scope : Scope
  Scope1 : Scope
  Scope2 : Scope
  Scope3 : Scope  NumInputPorts=2
  Scope4 : Scope  NumInputPorts=3
  Scope5 : Scope  NumInputPorts=2
  Scope6 : Scope  NumInputPorts=3
  Switch{,1..3} (4 alike) : Switch  Criteria=u2 > Threshold  SaturateOnIntegerOverflow=off  InputSameDT=off
  hip pitch : Scope
  knee : Scope
  smc : Subsystem
  InputFR : Outport  VectorParamsAs1DForOutWhenUnconnected=off
  InputFL : Outport  Port=2  VectorParamsAs1DForOutWhenUnconnected=off
  InputBR : Outport  Port=3  VectorParamsAs1DForOutWhenUnconnected=off
  InputBL : Outport  Port=4  VectorParamsAs1DForOutWhenUnconnected=off
  wires:
  refFL/1 -> LQR2 Controllers FL/1(ref), LQR Controllers FR1/1(ref)
  measBR/1 -> LQR2 Controllers BR/2(meas), LQR Controllers FR2/2(meas)
  refBR/1 -> LQR2 Controllers BR/1(ref), LQR Controllers FR2/1(ref)
  measFL/1 -> LQR2 Controllers FL/2(meas), LQR Controllers FR1/2(meas)
  refBL/1 -> LQR2 Controllers BL/1(ref), LQR Controllers FR3/1(ref)
  measBL/1 -> LQR2 Controllers BL/2(meas), LQR Controllers FR3/2(meas)
  Switch3/1 -> InputBL/1
  Switch2/1 -> InputBR/1
  Switch1/1 -> InputFL/1
  LQR Controllers FR/1(Input) -> Demux/1, Scope1/1, Switch/3
  LQR2 Controllers FR/1(Input) -> Demux1/1, Switch/1
  LQR Controllers FR1/1(Input) -> Switch1/3, Demux6/1
  LQR2 Controllers FL/1(Input) -> Switch1/1, Demux5/1
  LQR Controllers FR2/1(Input) -> Switch2/3
  LQR2 Controllers BR/1(Input) -> Switch2/1
  LQR Controllers FR3/1(Input) -> Switch3/3
  LQR2 Controllers BL/1(Input) -> Switch3/1
  [conFL] -> Scope6/3, Switch1/2
  [conBR] -> Switch2/2
  [conBL] -> Switch3/2
  [conFR] -> Scope/1, smc/Enable, Scope4/1, Scope2/1, NOT/1, Switch/2  "contact"
  NOT/1 -> Lqr/Enable
  Demux/1 -> Lqr/1(In1)
  Demux1/1 -> smc/1(In1)
  Lqr/1(Out1) -> Mux/1
  smc/1(Out1) -> Mux/2
  Mux/1 -> Scope4/2
  Switch/1 -> Demux2/1, InputFR/1
  Demux2/1 -> knee/1, Scope4/3  "control signal"
  Demux2/3 -> hip pitch/1
  measFR/1 -> Demux4/1, LQR2 Controllers FR/2(meas), LQR Controllers FR/2(meas)
  refFR/1 -> Demux3/1, LQR2 Controllers FR/1(ref), LQR Controllers FR/1(ref)
  Demux5/1 -> Scope6/1
  Demux6/1 -> Scope6/2
  Demux4/1 -> Scope3/2
  Demux3/3 -> Scope5/1
  Demux3/1 -> Scope3/1
  Demux4/3 -> Scope5/2

== system singlcontact_control_smc_lqr_mydimes_reaction/Walking Robot/NO CONTROLLER ==
  refFR : Inport
  refFL : Inport  Port=2
  measFR : Inport  Port=3
  measFL : Inport  Port=4
  measBL : Inport  Port=5
  measBR : Inport  Port=6
  refBR : Inport  Port=7
  refBL : Inport  Port=8
  Terminator{,1..3} (4 alike) : Terminator
  InputFR : Outport  VectorParamsAs1DForOutWhenUnconnected=off
  InputFL : Outport  Port=2  VectorParamsAs1DForOutWhenUnconnected=off
  InputBR : Outport  Port=3  VectorParamsAs1DForOutWhenUnconnected=off
  InputBL : Outport  Port=4  VectorParamsAs1DForOutWhenUnconnected=off
  wires:
  measBR/1 -> Terminator2/1
  measFL/1 -> Terminator1/1
  measBL/1 -> Terminator3/1
  refBL/1 -> InputBL/1
  refBR/1 -> InputBR/1
  refFL/1 -> InputFL/1
  refFR/1 -> InputFR/1
  measFR/1 -> Terminator/1

== system singlcontact_control_smc_lqr_mydimes_reaction/Walking Robot/Pid+Pid+reaction1 ==
  refFR : Inport
  refFL : Inport  Port=2
  measFR : Inport  Port=3
  measFL : Inport  Port=4
  measBL : Inport  Port=5
  measBR : Inport  Port=6
  refBR : Inport  Port=7
  refBL : Inport  Port=8
  Demux{,1..6} (7 alike) : Demux  Outputs=3
  Lqr : Subsystem
  Mux : Mux  Inputs=2
  NOT : Logic  Operator=NOT  IconShape=distinctive  AllPortsSameDT=off  OutDataTypeStr=boolean
  PID Controllers FR : Subsystem
  PID Controllers FR1 : Subsystem
  PID Controllers FR2 : Subsystem
  PID Controllers FR3 : Subsystem
  PID Controllers FR4 : Subsystem
  PID Controllers FR5 : Subsystem
  PID Controllers FR6 : Subsystem
  PID Controllers FR7 : Subsystem
  SMC Controllers FR1 : Subsystem  Commented=on
  SMC Controllers FR2 : Subsystem  Commented=on
  SMC Controllers FR3 : Subsystem  Commented=on
  Scope : Scope
  Scope1 : Scope
  Scope2 : Scope
  Scope3 : Scope  NumInputPorts=2
  Scope4 : Scope  NumInputPorts=3
  Scope5 : Scope  NumInputPorts=2
  Scope6 : Scope  NumInputPorts=3
  Switch{,1..3} (4 alike) : Switch  Criteria=u2 > Threshold  SaturateOnIntegerOverflow=off  InputSameDT=off
  hip pitch : Scope
  knee : Scope
  smc : Subsystem
  InputFR : Outport  VectorParamsAs1DForOutWhenUnconnected=off
  InputFL : Outport  Port=2  VectorParamsAs1DForOutWhenUnconnected=off
  InputBR : Outport  Port=3  VectorParamsAs1DForOutWhenUnconnected=off
  InputBL : Outport  Port=4  VectorParamsAs1DForOutWhenUnconnected=off
  wires:
  refFL/1 -> PID Controllers FR1/1(ref), PID Controllers FR5/1(ref)
  measBR/1 -> PID Controllers FR2/2(meas), PID Controllers FR6/2(meas)
  refBR/1 -> PID Controllers FR2/1(ref), PID Controllers FR6/1(ref)
  measFL/1 -> PID Controllers FR1/2(meas), PID Controllers FR5/2(meas)
  refBL/1 -> PID Controllers FR3/1(ref), PID Controllers FR7/1(ref)
  measBL/1 -> PID Controllers FR3/2(meas), PID Controllers FR7/2(meas)
  Switch3/1 -> InputBL/1
  Switch2/1 -> InputBR/1
  Switch1/1 -> InputFL/1
  PID Controllers FR/1(Input) -> Demux/1, Scope1/1, Switch/3
  PID Controllers FR4/1(Input) -> Demux1/1, Switch/1
  PID Controllers FR1/1(Input) -> Switch1/3, Demux6/1
  PID Controllers FR5/1(Input) -> Switch1/1, Demux5/1
  PID Controllers FR2/1(Input) -> Switch2/3
  PID Controllers FR6/1(Input) -> Switch2/1
  PID Controllers FR3/1(Input) -> Switch3/3
  PID Controllers FR7/1(Input) -> Switch3/1
  [conFL] -> Scope6/3, Switch1/2
  [conBR] -> Switch2/2
  [conBL] -> Switch3/2
  [conFR] -> Scope/1, smc/Enable, Scope4/1, Scope2/1, NOT/1, Switch/2  "contact"
  NOT/1 -> Lqr/Enable
  Demux/1 -> Lqr/1(In1)
  Demux1/1 -> smc/1(In1)
  Lqr/1(Out1) -> Mux/1
  smc/1(Out1) -> Mux/2
  Mux/1 -> Scope4/2
  Switch/1 -> Demux2/1, InputFR/1
  Demux2/1 -> knee/1, Scope4/3  "control signal"
  Demux2/3 -> hip pitch/1
  Demux4/3 -> Scope5/2
  Demux3/3 -> Scope5/1
  measFR/1 -> Demux4/1, PID Controllers FR/2(meas), PID Controllers FR4/2(meas)
  refFR/1 -> Demux3/1, PID Controllers FR/1(ref), PID Controllers FR4/1(ref)
  Demux3/1 -> Scope3/1
  Demux4/1 -> Scope3/2
  Demux5/1 -> Scope6/1
  Demux6/1 -> Scope6/2

== system singlcontact_control_smc_lqr_mydimes_reaction/Walking Robot/Robot Joint Controller ==
  note: 1) Add Subsystem or Model blocks as valid variant choices.
      | 2) You cannot connect blocks at this level. At simulation, connectivity is automatically
      | determined, based on the active variant and port name matching.
  refFR : Inport
  refFL : Inport  Port=2
  measFR : Inport  Port=3
  measFL : Inport  Port=4
  refFR1 : Inport  Port=5
  refFL1 : Inport  Port=6
  measBL : Inport  Port=7
  measBR : Inport  Port=8
  Motor : Subsystem  VariantControl=actuatorType == 3
  Torque : Subsystem  VariantControl=actuatorType == 2
  InputFR : Outport  VectorParamsAs1DForOutWhenUnconnected=off
  InputFL : Outport  Port=2  VectorParamsAs1DForOutWhenUnconnected=off
  InputBR1 : Outport  Port=3  VectorParamsAs1DForOutWhenUnconnected=off
  InputBL1 : Outport  Port=4  VectorParamsAs1DForOutWhenUnconnected=off
